simulink model "irec_simulink_model"  (R2016a)
settings: Solver=VariableStepAuto  StartTime=0.0  StopTime=10.0  RelTol=1e-3
libraries: aerolibatmos2 x2, aerolibasang x1
settings Model: Creator=Ian  LastModifiedBy=Ian

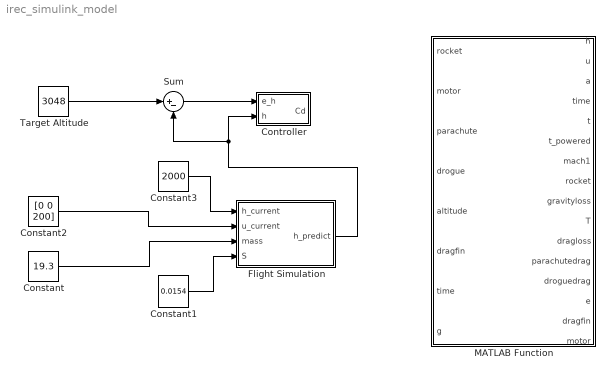
== system irec_simulink_model ==
  Constant : Constant  Value=19.3
  Constant1 : Constant  Value=0.0154
  Constant2 : Constant  Value=[0 0 200]
  Constant3 : Constant  Value=2000
  Controller : Subsystem
  Flight Simulation : Subsystem
  MATLAB Function : MATLAB Function  TreatAsAtomicUnit=on
  Sum : Sum  Inputs=|+-
  Target Altitude : Constant  Value=3048
  wires:
  Sum/1 -> Controller/1("e_h ")
  Target Altitude/1 -> Sum/1
  Constant/1 -> Flight Simulation/3(mass)
  Constant1/1 -> Flight Simulation/4(S)
  Constant2/1 -> Flight Simulation/2(u_current)
  Constant3/1 -> Flight Simulation/1(h_current)
  Flight Simulation/1(h_predict) -> Sum/2, Controller/2(h)

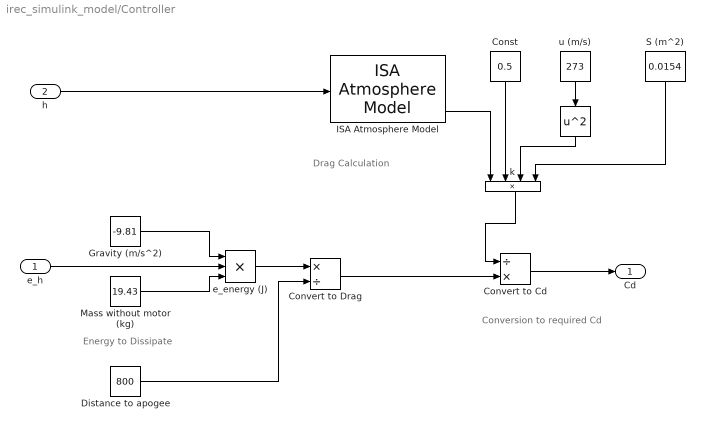
== system irec_simulink_model/Controller ==
  note: Conversion to required Cd
  note: Energy to Dissipate
  note: Drag Calculation
  "e_h " : Inport
  h : Inport  Port=2
  " " : Math  Operator=square  SaturateOnIntegerOverflow=on
  Const : Constant  Value=0.5
  Convert to Cd : Product  Inputs=/*
  Convert to Drag : Product  Inputs=*/
  Distance to apogee : Constant  Value=800
  Gravity (m/s^2) : Constant  Value=-9.81
  ISA Atmosphere Model : aerolibatmos2/ISA Atmosphere Model  custom=off  g=9.80665  gamma=1.4  R=287.0531  L=0.0065  h_trop=11000  h_strat=20000  rho0=1.225  P0=101325  T0=288.15  h0=0
  Mass without motor (kg) : Constant  Value=19.43
  S (m^2) : Constant  Value=0.0154
  e_energy (J) : Product  Inputs=3
  k : Product  Inputs=4
  u (m/s) : Constant  Value=273
  Cd : Outport
  wires:
  Mass without motor (kg)/1 -> e_energy (J)/3
  "e_h "/1 -> e_energy (J)/2
  Gravity (m/s^2)/1 -> e_energy (J)/1
  Distance to apogee/1 -> Convert to Drag/2
  e_energy (J)/1 -> Convert to Drag/1
  u (m/s)/1 -> " "/1
  ISA Atmosphere Model/4 -> k/1
  " "/1 -> k/3
  S (m^2)/1 -> k/4
  Const/1 -> k/2
  Convert to Cd/1 -> Cd/1
  h/1 -> ISA Atmosphere Model/1
  k/1 -> Convert to Cd/1
  Convert to Drag/1 -> Convert to Cd/2

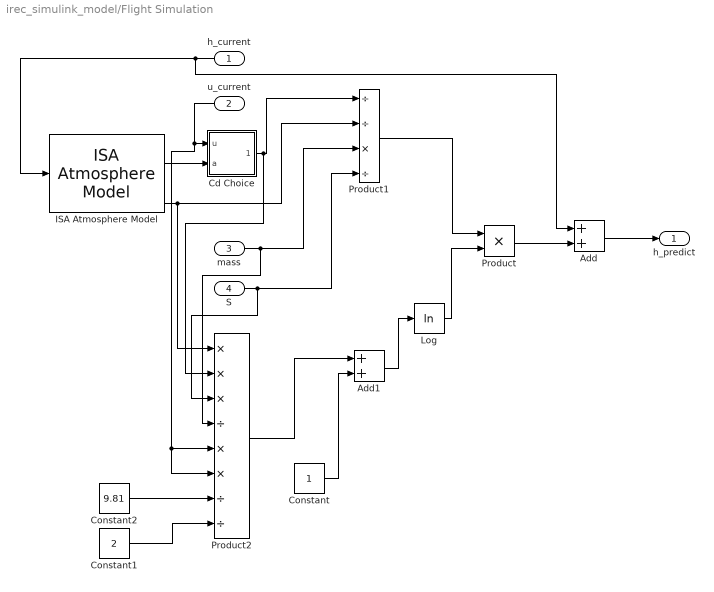
== system irec_simulink_model/Flight Simulation ==
  h_current : Inport
  u_current : Inport  Port=2
  mass : Inport  Port=3
  S : Inport  Port=4
  " Log" : Math  Operator=log  SaturateOnIntegerOverflow=on
  Add : Sum
  Add1 : Sum
  Cd Choice : Subsystem
  Constant : Constant
  Constant1 : Constant  Value=2
  Constant2 : Constant  Value=9.81
  ISA Atmosphere Model : aerolibatmos2/ISA Atmosphere Model  custom=off  g=9.80665  gamma=1.4  R=287.0531  L=0.0065  h_trop=11000  h_strat=20000  rho0=1.225  P0=101325  T0=288.15  h0=0
  Product : Product
  Product1 : Product  Inputs=//*/
  Product2 : Product  Inputs=***/**//
  h_predict : Outport
  wires:
  h_current/1 -> Add/1, ISA Atmosphere Model/1
  ISA Atmosphere Model/2 -> Cd Choice/2(a)
  u_current/1 -> Product2/6, Product2/5, Cd Choice/1(u)
  Product/1 -> Add/2
  Cd Choice/1(Cdeff) -> Product2/2, Product1/1
  ISA Atmosphere Model/4 -> Product1/2, Product2/1
  mass/1 -> Product2/4, Product1/3
  S/1 -> Product2/3, Product1/4
  " Log"/1 -> Product/2
  Product1/1 -> Product/1
  Constant/1 -> Add1/2
  Add1/1 -> " Log"/1
  Constant1/1 -> Product2/8
  Constant2/1 -> Product2/7
  Product2/1 -> Add1/1
  Add/1 -> h_predict/1

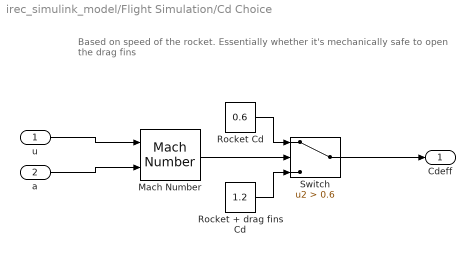
== system irec_simulink_model/Flight Simulation/Cd Choice ==
  note: Based on speed of the rocket. Essentially whether it's mechanically safe
      | to open the drag fins
  u : Inport
  a : Inport  Port=2
  Mach Number : aerolibasang/Mach Number
  Rocket + drag fins Cd : Constant  Value=1.2
  Rocket Cd : Constant  Value=0.6
  Switch : Switch  Criteria=u2 > Threshold  Threshold=0.6
  Cdeff : Outport
  wires:
  Mach Number/1 -> Switch/2
  Rocket Cd/1 -> Switch/1
  Rocket + drag fins Cd/1 -> Switch/3
  u/1 -> Mach Number/1
  a/1 -> Mach Number/2
  Switch/1 -> Cdeff/1

== matlab function irec_simulink_model/MATLAB Function ==
  data: rocket input; h output; motor input; parachute input; drogue input; altitude input; dragfin input; time input; g input; u output; a output; time output; t output; t_powered output; mach1 output; rocket output; gravityloss output; T output; dragloss output; parachutedrag output; droguedrag output; e output; dragfin output; motor output
% Drag Fin Sim
% This script runs a simulation of the rocket in flight with the goal of
% simulating the flight profile + drag fins
% Ian Gomez,  08/15/16
% Joan Creus, 08/16/16

% Primary Method:
% 1. Load the thrust data from ThrustCurve.org
% 2. Interpolate the data for more steps
% 3. Calculate change in mass from burnt prop
% 4. Calculate velocity from the combined impulse due to drag, gravity and thrust
% 5. Calculate altitude and acceleration from velocity
% https://spacegrant.carthage.edu/ojs/index.php/wsc/article/viewFile/23/23

function [h,u,a,time,t,t_powered,mach1,rocket,gravityloss,T,dragloss,...
    parachutedrag,droguedrag,e,dragfin,motor] = runSimulation(rocket,motor,...
    parachute,drogue,altitude,dragfin,time,g)

lam = cos(rocket.launch_angle.*pi./180); % launch angle multiplier for drag terms
drogue.deployed    = rocket.deploydrogue;
parachute.deployed = rocket.deployparachute;
parachute.deploy_h = altitude.launch_site + parachute.deploy_h;
parachute.S        = pi.*(parachute.d./2)^2; % m^2
drogue.S   = pi.*(drogue.d./2)^2;            % m^2
rocket.S   = pi.*(rocket.d./2).^2;           % m^2
parachute.S_normal = lam.*parachute.S;
drogue.S_normal    = lam.*drogue.S;
rocket.S_normal    = lam.*rocket.S;

% [motor,rocket,T,t_powered] = getMotorData(motor,rocket,time);

t = 0:time.step:time.end;                    % s

% Initialize gravity and mass for flight
m = rocket.drymass.*ones(1,length(t));       % kg
g = g.*ones(1,length(t));                    % m/s^2
% Vector initialization for speed
currentmomentum = zeros(1,length(t));
F = zeros(1,length(t)); u = zeros(1,length(t)); dragloss = zeros(1,length(t));
a = zeros(1,length(t)); h = zeros(1,length(t)); gravityloss = zeros(1,length(t));
parachutedrag = zeros(1,length(t)); droguedrag = zeros(1,length(t));
mach1 = zeros(1,length(t));
% Initial conditions
h(1) = altitude.launch_site; % m,   rocket is not at sea level
u(1) = 0;                    % m/s, rocket is stationary
m(1) = rocket.wetmass;       % kg,  rocket is full of prop

% Flight simulation
for i = 1:length(t)
    
    % if motor is on, lose mass
    if t(i) <= motor.burntime
        m(i+1) = m(i)-motor.mdotavg.*time.step;
        motor.burnout_h = h(i);
        motor.burnout_index = i;
    end
    
    % Drag calculation
    % The launch angle is taken into account here as well as the drag
    % multiplier for the drag fins
    [~,~,rho,mach1(i)] = getAtmoConditions(h(i));
    k = 0.5.*rocket.Cd.*rocket.S_normal.*rho;
    if (t(i)>dragfin.deploy_t && dragfin.deploy_t > 0 && u(i) > 0)
        k = dragfin.extra_drag_percent*k;
    end
    dragloss(i)        = k.*u(i).*abs(u(i));
    
    % Gravity loss and current momentum calculation
    % need to not allow gravity to move the rocket below starting altitude
    % if thrust doesn't take off right away
    gravityloss(i)     = m(i).*g(i);
    currentmomentum(i) = u(i).*m(i);
    
    % Recovery drag calculation
    % First if statement checks if the rocket is past the drogue deployment
    % speed and above parachute height
    % Second if statemnet checks if the rocket is below the parachute
    % deployment height
    if u(i) < drogue.deploy_u && h(i) > parachute.deploy_h && rocket.deploydrogue == 1
        droguedrag(i)    = 0.5.*drogue.Cd.*drogue.S_normal.*rho.*u(i).^2;
    elseif h(i) < parachute.deploy_h && u(i) < 0 && t(i) > 1 && rocket.deployparachute == 1
        parachutedrag(i) = 0.5.*parachute.Cd.*parachute.S_normal.*rho.*u(i).^2;
    end
    
    % Solve out forces on rocket
    if t(i) <= motor.burntime          % powered ascent
        F(i) = - gravityloss(i) - dragloss(i) + lam.*T(i);
    elseif u(i) > 0                    % coasting to apogee
        F(i) = - gravityloss(i) - dragloss(i);
    elseif 0 >= u(i) > drogue.deploy_u % descent
        F(i) = - gravityloss(i) + dragloss(i) + droguedrag(i)...
            + parachutedrag(i);
    end
    
    % Solve for new velocity and acceleration
    if(i < length(t)) % checks to not exceed index
        u(i+1)  = (1./m(i+1)).*(currentmomentum(i) + ((F(i)).*time.step));
        a(i)    = F(i)./m(i);
        h(i+1)  = trapz([0 time.step],[u(i) u(i+1)])+h(i);
    end
    
    % Store time at apogee and time at landing
    % u(i) < 0 is apogee; h(i) < 0 is landing
    if t(i) > 1 && h(i) >= (0 + altitude.launch_site)
        time.land = t(i);
    end
    if t(i) > 1 && u(i) > 0
        time.apogee = t(i);
        time.apogee_index = i;
    end
    
end

% Reset altitude for plotting. Air density already taken into account
h = h-altitude.launch_site;

% Store useful information
rocket.flight_time = time.land;
rocket.apogee = max(h);
rocket.burnout_h = motor.burnout_h;

% Energy calculations [J]
e.net  = rocket.drymass.*g(1).*rocket.apogee;
e.want = rocket.drymass.*g(end).*altitude.target;
e.diff = abs(e.net - e.want);
e.diff_perc = abs((e.net - e.want)/e.want);

if altitude.target > rocket.apogee % sign correction... because
    e.diff = -e.diff;
    e.diff_perc = -e.diff_perc;
end

% Drag fins deploy at time, t; finding the exact index of t allows us to
% find other important values at that time step
if dragfin.deploy_t > 0
    dragfin.deploy_index = getTimeIndex(t,dragfin.deploy_t,time.step);
    disp(strcat(strcat('Drag fins were deployed at ',...
        num2str(dragfin.deploy_t),'s')))
else % Pretend they deployed at some arbitrary time after burnout
    dragfin.dtab = 2; % deployment time after burnout
    dragfin.deploy_time = motor.burntime+dragfin.dtab;
    dragfin.deploy_index = getTimeIndex(t,dragfin.deploy_time,time.step);
    dragfin.deploy_h = h(dragfin.deploy_index); % m
    fprintf(strcat(strcat(...
        'Drag fins were not deployed, but if we did deploy at ',...
        num2str(dragfin.deploy_h),'m \n')))
    fields = {'extra_drag_percent','max_theta','dtab'};
    dragfin = rmfield(dragfin,fields); % removes extra fields from dragfin
end
dragfin.deploy_u = u(dragfin.deploy_index); % finds dragfin deploy u
dragfin.deploy_h = h(dragfin.deploy_index); % finds dragfin deploy h
dragfin.dist_to_apogee =  altitude.target - dragfin.deploy_h; % m
dragfin.extra_D_req = e.diff./dragfin.dist_to_apogee;         % N

end
